simulink model "MSFartoystyring"  (R2016b)
settings: Solver=ode45  StartTime=tstart  StopTime=tstop  RelTol=1e-3  EnableMultiTasking=on
values from neighbouring files (symbols this model uses):
  c = 1    [run.m]    (also in run_task_2.m; run_task_2_chi_feedback.m; run_task_2_psi_feedback.m)
  Kd = -53    [run.m]    (also in run_task_2.m; run_task_2_chi_feedback.m; run_task_2_psi_feedback.m = -100)
  Ki = -1.6e-3    (= -0.0016)    [run.m]    (also in run_task_2.m; run_task_2_chi_feedback.m; run_task_2_psi_feedback.m = -2e-05)
  Ki_u = 1e-2    (= 0.01)    [run.m]    (also in run_task_2.m; run_task_2_chi_feedback.m; run_task_2_psi_feedback.m)
  Kp = -8    [run.m]    (also in run_task_2.m; run_task_2_chi_feedback.m; run_task_2_psi_feedback.m = -1)
  Kp_u = 50    [run.m]    (also in run_task_2.m; run_task_2_chi_feedback.m; run_task_2_psi_feedback.m)
  psi0 = 0    [run.m]    (also in run_task_2.m; run_task_2_chi_feedback.m = deg2rad(60); run_task_2_psi_feedback.m = deg2rad(60))
  r0 = 0    [run.m]    (also in run_task_2.m; run_task_2_chi_feedback.m; run_task_2_psi_feedback.m)
  tsamp = 10    [run.m]    (also in run_task_2.m; run_task_2_chi_feedback.m; run_task_2_psi_feedback.m)
  u_reference_0 = 3    [run.m]    (also in run_task_2.m; run_task_2_chi_feedback.m; run_task_2_psi_feedback.m)
  u_reference_1 = 7    [run.m]    (also in run_task_2.m; run_task_2_chi_feedback.m; run_task_2_psi_feedback.m)
  v0 = [3 0]'    [run.m]    (also in run_task_2.m; run_task_2_chi_feedback.m = [6 63]'; run_task_2_psi_feedback.m = [6 63]')
undefined symbols (not defined in the file or in its folder): msfartoystyring
undefined symbols (not defined in the file): p0
settings Model: ExtModeAutoUpdateStatusClock=off  Creator=christh  LastModifiedBy=jonas
settings DataIOCC: LimitDataPoints=on  SaveFormat=Array  SignalLoggingSaveFormat=ModelDataLogs
settings OptimizationCC: ExpressionDepthLimit=2147483647  InitFltsAndDblsToZero=on  LifeSpan=inf
settings DebuggingCC: UnderspecifiedInitializationDetection=Classic  MergeDetectMultiDrivingBlocksExec=none  SolverPrmCheckMsg=warning  FcnCallInpInsideContextMsg=warning  StateNameClashWarn=warning  SFUnexpectedBacktrackingDiag=warning  SFNoUnconditionalDefaultTransitionDiag=warning  SFExecutionAtInitializationDiag=none
settings HardwareCC: ProdBitPerPointer=32  ProdBitPerSizeT=32  ProdBitPerPtrDiffT=32  ProdLargestAtomicFloat=None  ProdIntDivRoundTo=Undefined  ProdEndianess=Unspecified  ProdWordSize=32  ProdHWDeviceType=32-bit Generic
settings ModelReferenceCC: PropagateSignalLabelsOutOfModel=off
settings GRTTargetCC: TargetLangStandard=C89/C90 (ANSI)  GeneratePreprocessorConditionals=Disable all  CombineOutputUpdateFcns=off  GRTInterface=on
settings ConfigComp: CovMetricSettings=dw  CovHtmlReporting=on  CovSaveCumulativeToWorkspaceVar=on  CovSaveSingleToWorkspaceVar=on  CovExternalEMLEnable=off

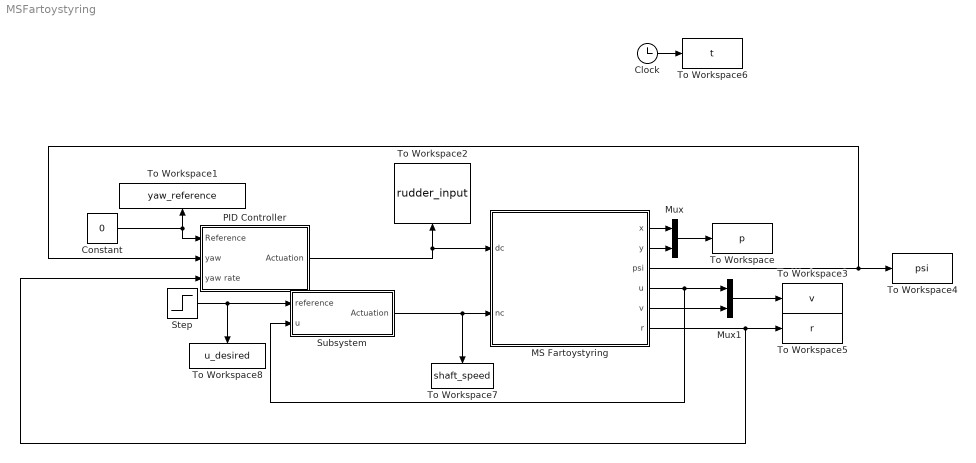
== system MSFartoystyring ==
  Clock : Clock
  Constant : Constant  Value=0
  MS Fartoystyring : Subsystem  mask(MS Fartoystyring for Assignment 3 G&C){x0=p0(1), y0=p0(2), u0=v0(1), v0=v0(2), psi0=psi0, r0=r0, c=c}
      mask prompts: x0 "x(t0) (m)"; y0 "y(t0) (m)"; u0 "u(t0) (m/s)"; v0 "v(t0) (m/s)"; psi0 "psi(t0) (rad)"; r0 "r(t0) (rad/s)"; c "current (0 or 1)"
      mask help:
      | Block corresponding to Figure 1 in the assignment text. Gives the response of the ship.
      |
      | The design speed of MS Fartoystyring is u=8.23 m/s.
      |
      | Input:
      | dc: commanded rudder (rad), dmax=25*pi/180
      | nc: commanded shaft speed (rad/s), nmax=85*2*pi/60
      |
      | Output:
      | x: north pos (m)
      | y: east pos (m)
      | u: surge (m/s)
      | v: sway (m/s)
      | psi: heading (rad)
      | r: yaw (rad/s)
      mask Help: Comments, bugs and help requests can be directed to the TA. Email on course website.
  Mux : Mux  Inputs=2
  Mux1 : Mux  Inputs=2
  PID Controller : Subsystem
  Step : Step  Time=1250  Before=u_reference_0  After=u_reference_1  SampleTime=tsamp
  Subsystem : Subsystem
  To Workspace : ToWorkspace  VariableName=p  SampleTime=tsamp
  To Workspace1 : ToWorkspace  VariableName=yaw_reference  SampleTime=tsamp
  To Workspace2 : ToWorkspace  VariableName=rudder_input  SampleTime=tsamp
  To Workspace3 : ToWorkspace  VariableName=v  SampleTime=tsamp
  To Workspace4 : ToWorkspace  VariableName=psi  SampleTime=tsamp
  To Workspace5 : ToWorkspace  VariableName=r  SampleTime=tsamp
  To Workspace6 : ToWorkspace  VariableName=t  SampleTime=tsamp
  To Workspace7 : ToWorkspace  VariableName=shaft_speed  SampleTime=tsamp
  To Workspace8 : ToWorkspace  VariableName=u_desired  SampleTime=tsamp
  wires:
  Clock/1 -> To Workspace6/1
  MS Fartoystyring/1(x) -> Mux/1
  MS Fartoystyring/2(y) -> Mux/2
  MS Fartoystyring/4(u) -> Subsystem/2("u "), Mux1/1
  MS Fartoystyring/5(v) -> Mux1/2
  Mux/1 -> To Workspace/1
  Mux1/1 -> To Workspace3/1
  MS Fartoystyring/3(psi) -> PID Controller/2("yaw "), To Workspace4/1
  MS Fartoystyring/6(r) -> PID Controller/3("yaw rate "), To Workspace5/1
  Subsystem/1("Actuation ") -> MS Fartoystyring/2(nc), To Workspace7/1
  Constant/1 -> PID Controller/1(Reference), To Workspace1/1
  PID Controller/1("Actuation ") -> To Workspace2/1, MS Fartoystyring/1(dc)
  Step/1 -> Subsystem/1("reference "), To Workspace8/1

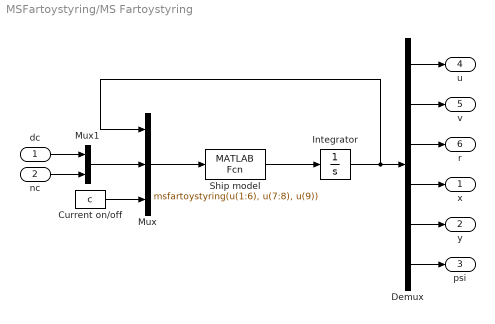
== system MSFartoystyring/MS Fartoystyring ==
  dc : Inport
  nc : Inport  Port=2
  Current on/off : Constant  Value=c
  Demux : Demux  Outputs=6
  Integrator : Integrator  InitialCondition=[u0 v0 r0 x0 y0 psi0]'
  Mux : Mux  Inputs=3
  Mux1 : Mux  Inputs=2
  Ship model : MATLABFcn  MATLABFcn=msfartoystyring(u(1:6), u(7:8), u(9))  OutputDimensions=6
  x : Outport
  y : Outport  Port=2
  psi : Outport  Port=3
  u : Outport  Port=4
  v : Outport  Port=5
  r : Outport  Port=6
  wires:
  Integrator/1 -> Mux/1, Demux/1
  Mux1/1 -> Mux/2
  dc/1 -> Mux1/1
  nc/1 -> Mux1/2
  Demux/1 -> u/1
  Demux/2 -> v/1
  Demux/3 -> r/1
  Demux/4 -> x/1
  Demux/5 -> y/1
  Demux/6 -> psi/1
  Current on/off/1 -> Mux/3
  Ship model/1 -> Integrator/1
  Mux/1 -> Ship model/1

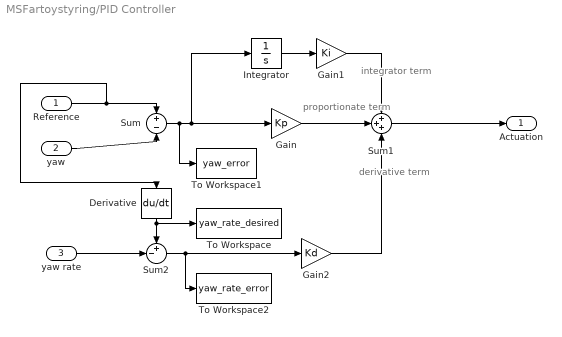
== system MSFartoystyring/PID Controller ==
  note: derivative
      | term
  note: proportionate term
  note: integrator
      | term
  Reference : Inport
  "yaw " : Inport  Port=2
  "yaw rate " : Inport  Port=3
  Derivative : Derivative
  Gain : Gain  Gain=Kp
  Gain1 : Gain  Gain=Ki
  Gain2 : Gain  Gain=Kd
  Integrator : Integrator
  Sum : Sum  Inputs=+|-
  Sum1 : Sum  Inputs=+++
  Sum2 : Sum  Inputs=+-|
  To Workspace : ToWorkspace  VariableName=yaw_rate_desired  SampleTime=tsamp
  To Workspace1 : ToWorkspace  VariableName=yaw_error  SampleTime=tsamp
  To Workspace2 : ToWorkspace  VariableName=yaw_rate_error  SampleTime=tsamp
  "Actuation " : Outport
  wires:
  Reference/1 -> Derivative/1, Sum/1
  "yaw "/1 -> Sum/2
  Sum/1 -> To Workspace1/1, Integrator/1, Gain/1
  Sum1/1 -> "Actuation "/1
  Gain/1 -> Sum1/2
  Derivative/1 -> To Workspace/1, Sum2/1
  "yaw rate "/1 -> Sum2/2
  Sum2/1 -> To Workspace2/1, Gain2/1
  Gain2/1 -> Sum1/3
  Gain1/1 -> Sum1/1
  Integrator/1 -> Gain1/1

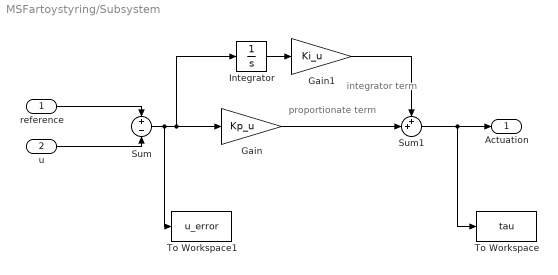
== system MSFartoystyring/Subsystem ==
  note: proportionate term
  note: integrator
      | term
  "reference " : Inport
  "u " : Inport  Port=2
  Gain : Gain  Gain=Kp_u
  Gain1 : Gain  Gain=Ki_u
  Integrator : Integrator
  Sum : Sum  Inputs=+|-
  Sum1 : Sum  Inputs=++|
  To Workspace : ToWorkspace  VariableName=tau  SaveFormat=Timeseries  SampleTime=-1
  To Workspace1 : ToWorkspace  VariableName=u_error  SampleTime=tsamp
  "Actuation " : Outport
  wires:
  "reference "/1 -> Sum/1
  "u "/1 -> Sum/2
  Sum/1 -> To Workspace1/1, Integrator/1, Gain/1
  Sum1/1 -> To Workspace/1, "Actuation "/1
  Gain/1 -> Sum1/2
  Gain1/1 -> Sum1/1
  Integrator/1 -> Gain1/1
